simulink subsystem "MTQ"  (R2025b)
settings: Solver=VariableStepAuto  StartTime=0.0  StopTime=10.0  RelTol=1e-3
model mask{mtqMagneticGain=0, mtqResistance=0, mtqMaxVoltage=0}
  mask prompts: mtqMagneticGain "Magnetic gain [Am2A-1]"; mtqResistance "Electrical resistance [Ohm]"; mtqMaxVoltage "Maximum voltage [V]"
settings Model: Creator=antoniohernandez-rodiciomateos  LastModifiedBy=antoniohernandez-rodiciomateos

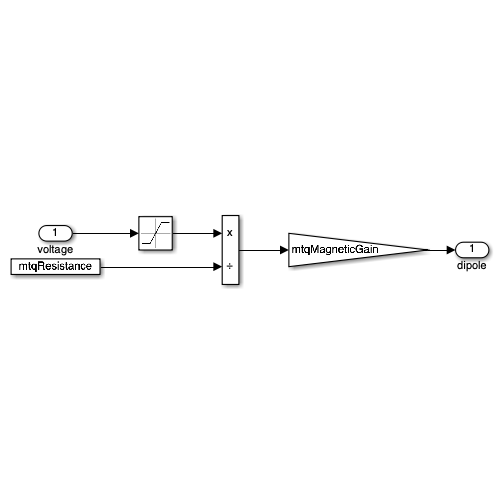
[thumbnail: Simulink's stored preview of the top-level diagram]
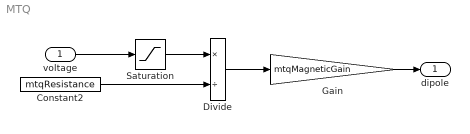
== system MTQ ==
  voltage : Inport  OutDataTypeStr=double  PortDimensions=[1 1]
  Constant2 : Constant  Value=mtqResistance
  Divide : Product  Inputs=*/
  Gain : Gain  Gain=mtqMagneticGain
  Saturation : Saturate  UpperLimit=mtqMaxVoltage  LowerLimit=0
  dipole : Outport  OutDataTypeStr=double  PortDimensions=[1 1]
  wires:
  voltage/1 -> Saturation/1
  Saturation/1 -> Divide/1
  Constant2/1 -> Divide/2
  Divide/1 -> Gain/1
  Gain/1 -> dipole/1
